simulink model "PECT08"  (R2015b)
settings: Solver=FixedStepAuto  StartTime=0.0  StopTime=100  RelTol=1e-3
undefined symbols (not defined in the file): PDRref, sigbuilder_block
libraries: slrtlib x13, xpcnilib x11, simulink x9, dspfdesign x7, simulink_extras x1
(part 2 of 3)

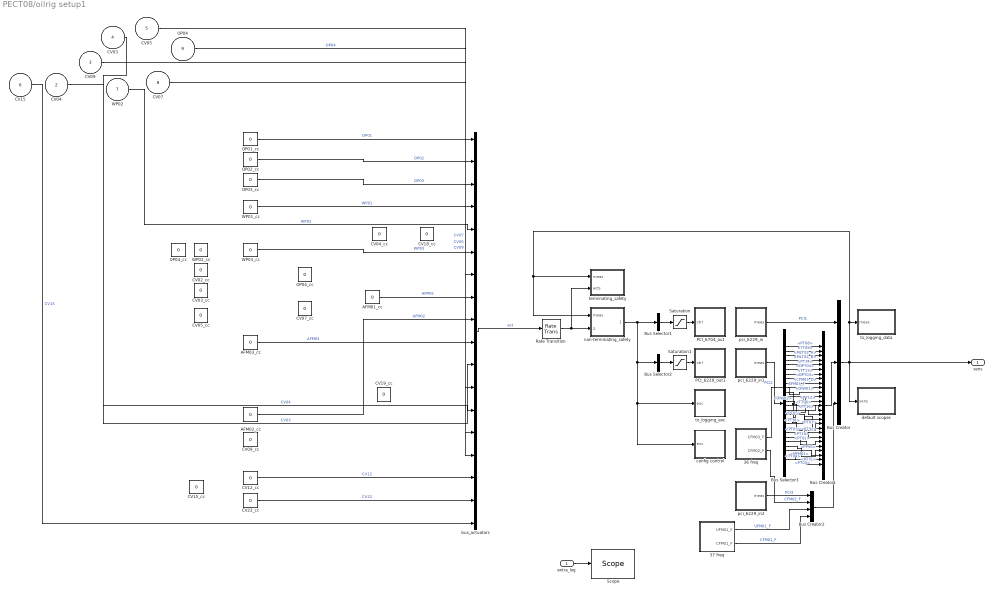
== system PECT08/oilrig setup1 ==
  extra_log : Inport
  CV04 : Inport  Port=2
  CV09 : Inport  Port=3
  CV03 : Inport  Port=4
  CV05 : Inport  Port=5
  CV15 : Inport  Port=6
  WP02 : Inport  Port=7
  CV07 : Inport  Port=8
  OP04 : Inport  Port=9
  0P04_cc : Constant  Value=0
  36 freq : Subsystem  mask{subsystem=[3,6]}
      mask init:
      | sensors = evalin('base','sensors');
      | 
      | subsystem = sprintf('[%d,%d]', subsystem(1), subsystem(2));
      | 
      | freqin = sensors(strcmp(subsystem,{sensors.PCIslot})&(strcmp('FI|0-10000Hz',{sensors.Type})));
      | if ~isempty(freqin)
      |     disp(['PCI slot ' subsystem ' loading']);
      | else
      |     error('There are no frequency inputs in the given card'); 
      | end
  37 freq : Subsystem  mask{subsystem=[3,7]}
      mask init: same as PECT08/oilrig setup1/36 freq
  AFM01_cc : Constant  Value=0
  AFM02_cc : Constant  Value=0
  AFM03_cc : Constant  Value=0
  Bus Creator : BusCreator  Inputs=3
  Bus Creator1 : BusCreator  Inputs=27
  Bus Creator2 : BusCreator  Inputs=4
  Bus Selector1 : BusSelector  OutputSignals=OP01,OP02,OP03,WP01,WP02,OP04,AFM01,AFM02,AFM03,CV03,CV04,CV09,CV05,CV12,CV22,CV15  OutputAsBus=on
  Bus Selector2 : BusSelector  OutputSignals=WP03,CV07  OutputAsBus=on
  Bus Selector3 : BusSelector  OutputSignals=PT08,TT09,MLT02_A,MLT02_B,PT14,DPT04,TT13,DPT03,CFM03_D,OIW01,OIW02,PT12,PT16,TT06,PT05,PT07,PT10,TT11,PT32,TT03,PT15,PT02,PT31,MFM01,PT03,TT04
  CV02_cc : Constant  Value=0
  CV03_cc : Constant  Value=0
  CV04_cc : Constant  Value=0
  CV05_cc : Constant  Value=0
  CV07_cc : Constant  Value=0
  CV09_cc : Constant  Value=0
  CV12_cc : Constant  Value=0
  CV15_cc : Constant  Value=0
  CV18_cc : Constant  Value=0
  CV19_cc : Constant  Value=0
  CV22_cc : Constant  Value=0
  OP01_cc : Constant  Value=0
  OP02_cc : Constant  Value=0
  OP03_cc : Constant  Value=0
  OP04_cc : Constant  Value=0
  PCI_6229_out1 : Subsystem  mask(Actuator output){subsystem=[3,5]}
      mask help: Converts and outputs actuators connected to one PCI-6229 card.
      mask init:
      | %%Get analog channels
      | actuators = evalin('base','actuators');
      | 
      | subsystem = sprintf('[%d,%d]', subsystem(1), subsystem(2));
      | 
      | analogout = actuators(strcmp(subsystem,{actuators.PCIslot}));
      | 
      | src_block = find_system(gcb, 'LookUnderMasks', 'on','Name', 'DA_sink');
      | maskObj = Simulink.Mask.get(src_block{1});
      | 
      | if(isempty(analogout))
      |    error('There are no analog outputs in the given card'); 
      | end
      | 
      | maskObj.Parameters(1,5).Value = subsystem;
      | maskObj.Parameters(1,1).Value = mat2str([analogout.Chan]+1);
      | Simulink.Block.eval(src_block{1});
      | 
      | %Find block
      | transform_blk = find_system(gcb, 'LookUnderMasks', 'on','Name', 'transform');
      | 
      | outputnames = {analogout.ElementName};
      | outputs = strjoin(outputnames,',');
      | 
      | sigcount = numel(outputnames);
      | sigstring = num2str(sigcount);
      | 
      | %Transform block
      | transform_blk = find_system(gcb, 'LookUnderMasks', 'on','Name', 'transform');
      | lines{1}=['function [' outputs ']  = fcn(u,gain,offset)'];
      | lines{2}='   y = u.*gain-offset;';
      | for i=1:numel(outputnames)
      |    %start at 4
      |    lines{2+i} = [ outputnames{i} ' = y(' num2str(i) ');'];
      | end
      | outputscript = strjoin(lines,'\n');
      | matlabfunctionfromstring(transform_blk{1}, outputscript);
      | Simulink.Block.eval(transform_blk{1});
      | 
      | %Delete lines
      | connections = find_system(gcb,'findall','on','LookUnderMasks', 'on','SearchDepth', 1,'type','line');
      | delete_line(connections);
      | 
      | for i=1:numel(outputnames)
      |    add_line(gcb,['transform/' num2str(i) ],['DA_sink/' num2str(i)],'autorouting','on');
      | end
      | 
      | %Transform block
      | add_line(gcb,'ctrl/1','transform/1','autorouting','on')
      | add_line(gcb,'gain/1','transform/2','autorouting','on')
      | add_line(gcb,'offset/1','transform/3','autorouting','on')
      | 
      | gain = [analogout.Gain]';
      | offset = [analogout.Offset]';
      mask DialogControl Control2 Prompt: Subsystem description struct
  PCI_6704_out : Subsystem  mask(Actuator output){subsystem=[3,4]}
      mask help: Converts and outputs actuators connected to one PCI-6229 card.
      mask init:
      | %%Get analog channels
      | actuators = evalin('base','actuators');
      | 
      | subsystem = sprintf('[%d,%d]', subsystem(1), subsystem(2));
      | 
      | analogout = actuators(strcmp(subsystem,{actuators.PCIslot}));
      | 
      | src_block = find_system(gcb, 'LookUnderMasks', 'on','Name', 'DA_sink');
      | maskObj = Simulink.Mask.get(src_block{1});
      | 
      | if(isempty(analogout))
      |    error('There are no analog outputs in the given card'); 
      | end
      | 
      | maskObj.Parameters(1,3).Value = subsystem;
      | maskObj.Parameters(1,1).Value = mat2str([analogout.Chan]+1);
      | Simulink.Block.eval(src_block{1});
      | 
      | %Find block
      | transform_blk = find_system(gcb, 'LookUnderMasks', 'on','Name', 'transform');
      | 
      | outputnames = {analogout.ElementName};
      | outputs = strjoin(outputnames,',');
      | 
      | sigcount = numel(outputnames);
      | sigstring = num2str(sigcount);
      | 
      | %Transform block
      | transform_blk = find_system(gcb, 'LookUnderMasks', 'on','Name', 'transform');
      | lines{1}=['function [' outputs ']  = fcn(u,gain,offset)'];
      | lines{2}='   y = u.*gain-offset;';
      | for i=1:numel(outputnames)
      |    %start at 4
      |    lines{2+i} = [ outputnames{i} ' = y(' num2str(i) ');'];
      | end
      | outputscript = strjoin(lines,'\n');
      | matlabfunctionfromstring(transform_blk{1}, outputscript);
      | Simulink.Block.eval(transform_blk{1});
      | 
      | %Delete lines
      | connections = find_system(gcb,'findall','on','LookUnderMasks', 'on','SearchDepth', 1,'type','line');
      | delete_line(connections);
      | 
      | for i=1:numel(outputnames)
      |    add_line(gcb,['transform/' num2str(i) ],['DA_sink/' num2str(i)],'autorouting','on');
      | end
      | 
      | %Transform block
      | add_line(gcb,'ctrl/1','transform/1','autorouting','on')
      | add_line(gcb,'gain/1','transform/2','autorouting','on')
      | add_line(gcb,'offset/1','transform/3','autorouting','on')
      | 
      | gain = [analogout.Gain]';
      | offset = [analogout.Offset]';
      mask DialogControl Control2 Prompt: Subsystem description struct
  Rate Transition : RateTransition
  Saturation : Saturate  UpperLimit=1  LowerLimit=0
  Saturation1 : Saturate  UpperLimit=1  LowerLimit=0
  "Scope " : slrtlib/Displays and Logging/Scope   scopeno=3  scopetype=Host  autostart=on  viewmode=Graphical sliding  formatstr='%15.6f'  grid=on  ylimits=[1.5,2.5]  nosamples=300  noprepostsamples=0  interleave=1  triggermode=FreeRun  triggersignal=1  trigsignalfromport=off  triggerlevel=0.0  triggerslope=Either  triggerscope=1  triggersample=0  filename=data.dat  mode=Lazy  writesize=512  autorestart=off  dynamicfilemode=off  maxwritefilesize=512*1024^2
  WP01_cc : Constant  Value=0
  WP02_cc : Constant  Value=0
  WP03_cc : Constant  Value=0
  bus_actuators : BusCreator  Inputs=18
  config control : Subsystem
  default scopes : Subsystem
  non-terminating_safety : Subsystem
  pci_6229_in : Subsystem  mask(Sensor reader){subsystem=[3,5]}
      mask help: Reads and converts sensors connected to one PCI-6229 card.
      mask init:
      | %%Get analog channels
      | sensors = evalin('base','sensors');
      | 
      | subsystem = sprintf('[%d,%d]', subsystem(1), subsystem(2));
      | 
      | analogin = sensors(strcmp(subsystem,{sensors.PCIslot})&(strcmp('VI|0-10V',{sensors.Type})|strcmp('VI|2-10V',{sensors.Type})|strcmp('CI|4-20mA',{sensors.Type})));
      | if ~isempty(analogin)
      |     disp(['PCI slot ' subsystem ' loading']);
      | else
      |     error('There are no analog inputs in the given card'); 
      | end
      | 
      | 
      | %%Find source (ADC) block
      | src_block = find_system(gcb, 'LookUnderMasks', 'on','Name', 'src');
      | maskObj = Simulink.Mask.get(src_block{1});
      | 
      | maskObj.Parameters(1,6).Value = subsystem;
      | maskObj.Parameters(1,1).Value = mat2str([analogin.Chan]+1);
      | Simulink.Block.eval(src_block{1});
      | 
      | %Find block
      | transform_blk = find_system(gcb, 'LookUnderMasks', 'on','Name', 'transform');
      | 
      | outputnames = {analogin.ElementName};
      | outputs = strjoin(outputnames,',');
      | 
      | sigcount = numel(outputnames);
      | sigstring = num2str(sigcount);
      | 
      | %Transform block
      | transform_blk = find_system(gcb, 'LookUnderMasks', 'on','Name', 'transform');
      | lines{1}=['function [' outputs ']  = fcn(u,gain,offset)'];
      | lines{2}='   y = u.*gain-offset;';
      | for i=1:numel(outputnames)
      |    %start at 4
      |    lines{2+i} = [ outputnames{i} ' = y(' num2str(i) ');'];
      | end
      | outputscript = strjoin(lines,'\n');
      | matlabfunctionfromstring(transform_blk{1}, outputscript);
      | Simulink.Block.eval(transform_blk{1});
      | 
      | %Delete lines
      | connections = find_system(gcb,'findall','on','LookUnderMasks', 'on','SearchDepth', 1,'type','line');
      | delete_line(connections);
      | 
      | %Mux block
      | mux_blk = find_system(gcb, 'LookUnderMasks', 'on','Name', 'mux');
      | set_param(mux_blk{1},'Inputs', sigstring);
      | Simulink.Block.eval(mux_blk{1});
      | 
      | %Bus block
      | bus_blk = find_system(gcb, 'LookUnderMasks', 'on','Name', 'bus');
      | set_param(bus_blk{1},'Inputs', sigstring);
      | Simulink.Block.eval(bus_blk{1});
      | 
      | for i=1:numel(outputnames)
      |    add_line(gcb,['src/' num2str(i) ],['mux/' num2str(i)],'autorouting','on');
      |    add_line(gcb,['transform/' num2str(i) ],['bus/' num2str(i)],'autorouting','on');
      | end
      | 
      | %Lines to bus block
      | p = get_param(transform_blk, 'PortHandles');
      | l = get_param(p{1}.Outport,'Line');
      | 
      | for i=1:numel(outputnames)
      |    set_param(l{i},'Name',outputnames{i}) 
      | end
      | 
      | %Transform block
      | add_line(gcb,'mux/1','transform/1','autorouting','on')
      | add_line(gcb,'gain/1','transform/2','autorouting','on')
      | add_line(gcb,'offset/1','transform/3','autorouting','on')
      | add_line(gcb,'bus/1','meas/1','autorouting','on')
      | 
      | gain = [analogin.Gain]';
      | offset = [analogin.Offset]';
      mask DialogControl Control2 Prompt: Subsystem description struct
  pci_6229_in1 : Subsystem  mask(Sensor reader){subsystem=[3,6]}
      mask help: Reads and converts sensors connected to one PCI-6229 card.
      mask init:
      | %%Get analog channels
      | sensors = evalin('base','sensors');
      | 
      | subsystem = sprintf('[%d,%d]', subsystem(1), subsystem(2));
      | 
      | freqin = sensors(strcmp(subsystem,{sensors.PCIslot})&(strcmp('FI|0-10000Hz',{sensors.Type})));
      | if ~isempty(freqin)
      |     disp(['PCI slot ' subsystem ' loading']);
      | else
      |     error('There are no frequency inputs in the given card'); 
      | end
      | 
      | analogin = sensors(strcmp(subsystem,{sensors.PCIslot})&(strcmp('VI|0-10V',{sensors.Type})|strcmp('VI|2-10V',{sensors.Type})|strcmp('CI|4-20mA',{sensors.Type})));
      | if ~isempty(analogin)
      |     disp(['PCI slot ' subsystem ' loading']);
      | else
      |     error('There are no analog inputs in the given card'); 
      | end
      | 
      | 
      | %%Find source (ADC) block
      | src_block = find_system(gcb, 'LookUnderMasks', 'on','Name', 'src');
      | maskObj = Simulink.Mask.get(src_block{1});
      | 
      | maskObj.Parameters(1,6).Value = subsystem;
      | maskObj.Parameters(1,1).Value = mat2str([analogin.Chan]+1);
      | Simulink.Block.eval(src_block{1});
      | 
      | %Find block
      | transform_blk = find_system(gcb, 'LookUnderMasks', 'on','Name', 'transform');
      | 
      | outputnames = {analogin.ElementName};
      | outputs = strjoin(outputnames,',');
      | 
      | sigcount = numel(outputnames);
      | sigstring = num2str(sigcount);
      | 
      | %Transform block
      | transform_blk = find_system(gcb, 'LookUnderMasks', 'on','Name', 'transform');
      | lines{1}=['function [' outputs ']  = fcn(u,gain,offset)'];
      | lines{2}='   y = u.*gain-offset;';
      | for i=1:numel(outputnames)
      |    %start at 4
      |    lines{2+i} = [ outputnames{i} ' = y(' num2str(i) ');'];
      | end
      | outputscript = strjoin(lines,'\n');
      | matlabfunctionfromstring(transform_blk{1}, outputscript);
      | Simulink.Block.eval(transform_blk{1});
      | 
      | %Delete lines
      | connections = find_system(gcb,'findall','on','LookUnderMasks', 'on','SearchDepth', 1,'type','line');
      | delete_line(connections);
      | 
      | %Mux block
      | mux_blk = find_system(gcb, 'LookUnderMasks', 'on','Name', 'mux');
      | set_param(mux_blk{1},'Inputs', sigstring);
      | Simulink.Block.eval(mux_blk{1});
      | 
      | %Bus block
      | bus_blk = find_system(gcb, 'LookUnderMasks', 'on','Name', 'bus');
      | set_param(bus_blk{1},'Inputs', sigstring);
      | Simulink.Block.eval(bus_blk{1});
      | 
      | for i=1:numel(outputnames)
      |    add_line(gcb,['src/' num2str(i) ],['mux/' num2str(i)],'autorouting','on');
      |    add_line(gcb,['transform/' num2str(i) ],['bus/' num2str(i)],'autorouting','on');
      | end
      | 
      | %Lines to bus block
      | p = get_param(transform_blk, 'PortHandles');
      | l = get_param(p{1}.Outport,'Line');
      | 
      | for i=1:numel(outputnames)
      |    set_param(l{i},'Name',outputnames{i}) 
      | end
      | 
      | %Transform block
      | add_line(gcb,'mux/1','transform/1','autorouting','on')
      | add_line(gcb,'gain/1','transform/2','autorouting','on')
      | add_line(gcb,'offset/1','transform/3','autorouting','on')
      | add_line(gcb,'bus/1','meas/1','autorouting','on')
      | 
      | gain = [analogin.Gain]';
      | offset = [analogin.Offset]';
      mask DialogControl Control2 Prompt: Subsystem description struct
  pci_6229_in2 : Subsystem  mask(Sensor reader){subsystem=[3,7]}
      mask help: Reads and converts sensors connected to one PCI-6229 card.
      mask init:
      | %%Get analog channels
      | sensors = evalin('base','sensors');
      | 
      | subsystem = sprintf('[%d,%d]', subsystem(1), subsystem(2));
      | 
      | analogin = sensors(strcmp(subsystem,{sensors.PCIslot})&(strcmp('VI|0-10V',{sensors.Type})|strcmp('VI|2-10V',{sensors.Type})|strcmp('CI|4-20mA',{sensors.Type})));
      | if ~isempty(analogin)
      |     disp(['PCI slot ' subsystem ' loading']);
      | else
      |     error('There are no analog inputs in the given card'); 
      | end
      | 
      | freqin = sensors(strcmp(subsystem,{sensors.PCIslot})&(strcmp('FI|0-10000Hz',{sensors.Type})));
      | if ~isempty(freqin)
      |     disp(['PCI slot ' subsystem ' loading']);
      | else
      |     error('There are no analog inputs in the given card'); 
      | end
      | 
      | 
      | 
      | %%Find source (ADC) block
      | src_block = find_system(gcb, 'LookUnderMasks', 'on','Name', 'src');
      | maskObj = Simulink.Mask.get(src_block{1});
      | 
      | maskObj.Parameters(1,6).Value = subsystem;
      | maskObj.Parameters(1,1).Value = mat2str([analogin.Chan]+1);
      | Simulink.Block.eval(src_block{1});
      | 
      | %Find block
      | transform_blk = find_system(gcb, 'LookUnderMasks', 'on','Name', 'transform');
      | 
      | outputnames = {analogin.ElementName};
      | outputs = strjoin(outputnames,',');
      | 
      | sigcount = numel(outputnames);
      | sigstring = num2str(sigcount);
      | 
      | %Transform block
      | transform_blk = find_system(gcb, 'LookUnderMasks', 'on','Name', 'transform');
      | lines{1}=['function [' outputs ']  = fcn(u,gain,offset)'];
      | lines{2}='   y = u.*gain-offset;';
      | for i=1:numel(outputnames)
      |    %start at 4
      |    lines{2+i} = [ outputnames{i} ' = y(' num2str(i) ');'];
      | end
      | outputscript = strjoin(lines,'\n');
      | matlabfunctionfromstring(transform_blk{1}, outputscript);
      | Simulink.Block.eval(transform_blk{1});
      | 
      | %Delete lines
      | connections = find_system(gcb,'findall','on','LookUnderMasks', 'on','SearchDepth', 1,'type','line');
      | delete_line(connections);
      | 
      | %Mux block
      | mux_blk = find_system(gcb, 'LookUnderMasks', 'on','Name', 'mux');
      | set_param(mux_blk{1},'Inputs', sigstring);
      | Simulink.Block.eval(mux_blk{1});
      | 
      | %Bus block
      | bus_blk = find_system(gcb, 'LookUnderMasks', 'on','Name', 'bus');
      | set_param(bus_blk{1},'Inputs', sigstring);
      | Simulink.Block.eval(bus_blk{1});
      | 
      | for i=1:numel(outputnames)
      |    add_line(gcb,['src/' num2str(i) ],['mux/' num2str(i)],'autorouting','on');
      |    add_line(gcb,['transform/' num2str(i) ],['bus/' num2str(i)],'autorouting','on');
      | end
      | 
      | %Lines to bus block
      | p = get_param(transform_blk, 'PortHandles');
      | l = get_param(p{1}.Outport,'Line');
      | 
      | for i=1:numel(outputnames)
      |    set_param(l{i},'Name',outputnames{i}) 
      | end
      | 
      | %Transform block
      | add_line(gcb,'mux/1','transform/1','autorouting','on')
      | add_line(gcb,'gain/1','transform/2','autorouting','on')
      | add_line(gcb,'offset/1','transform/3','autorouting','on')
      | add_line(gcb,'bus/1','meas/1','autorouting','on')
      | 
      | gain = [analogin.Gain]';
      | offset = [analogin.Offset]';
      mask DialogControl Control2 Prompt: Subsystem description struct
  terminating_safety : Subsystem
  to_logging_data : Subsystem
  to_logging_exc : Subsystem
  sens : Outport
  wires:
  non-terminating_safety/1(acts_out) -> config control/1(exc), to_logging_exc/1(exc), Bus Selector2/1, Bus Selector1/1
  pci_6229_in/1(meas) -> Bus Creator/1  "PCI1"
  Bus Selector3/2 -> Bus Creator1/2  "<TT09>"
  Bus Selector3/3 -> Bus Creator1/3  "<MLT02_A>"
  Bus Selector3/9 -> Bus Creator1/9  "<CFM03_D>"
  Bus Selector3/24 -> Bus Creator1/25  "<MFM01>"
  Bus Selector3/25 -> Bus Creator1/26  "<PT03>"
  Bus Selector3/21 -> Bus Creator1/22  "<PT15>"
  pci_6229_in2/1(meas) -> Bus Creator2/1  "PCI3"
  bus_actuators/1 -> Rate Transition/1  "act"
  Rate Transition/1 -> terminating_safety/2(acts), non-terminating_safety/2(acts_in)
  Bus Selector1/1 -> Saturation/1
  Bus Selector3/4 -> Bus Creator1/4  "<MLT02_B>"
  Bus Selector3/14 -> Bus Creator1/15  "<TT06>"
  Bus Selector3/26 -> Bus Creator1/27  "<TT04>"
  Bus Selector3/23 -> Bus Creator1/24  "<PT31>"
  Bus Selector3/16 -> Bus Creator1/17  "<PT07>"
  Bus Selector3/22 -> Bus Creator1/23  "<PT02>"
  Bus Selector3/20 -> Bus Creator1/21  "<TT03>"
  Bus Selector3/18 -> Bus Creator1/19  "<TT11>"
  Bus Selector2/1 -> Saturation1/1
  pci_6229_in1/1(meas) -> Bus Selector3/1  "PCI2"
  Bus Selector3/1 -> Bus Creator1/1  "<PT08>"
  Bus Selector3/5 -> Bus Creator1/5  "<PT14>"
  Bus Selector3/7 -> Bus Creator1/7  "<TT13>"
  Bus Selector3/19 -> Bus Creator1/20  "<PT32>"
  Bus Selector3/6 -> Bus Creator1/6  "<DPT04>"
  37 freq/1(UFM01_F) -> Bus Creator2/3  "UFM01_F"
  Bus Selector3/17 -> Bus Creator1/18  "<PT10>"
  Bus Selector3/8 -> Bus Creator1/8  "<DPT03>"
  Bus Creator1/1 -> Bus Creator/2
  Bus Selector3/13 -> Bus Creator1/14  "<PT16>"
  Bus Creator/1 -> sens/1, non-terminating_safety/1(meas), terminating_safety/1(meas), to_logging_data/1(meas), default scopes/1(sens)
  36 freq/1(CFM03_F) -> Bus Creator1/10  "CFM03_F"
  Bus Selector3/15 -> Bus Creator1/16  "<PT05>"
  36 freq/2(CFM02_F) -> Bus Creator2/2  "CFM02_F"
  Saturation1/1 -> PCI_6229_out1/1(ctrl)
  Saturation/1 -> PCI_6704_out/1(ctrl)
  Bus Creator2/1 -> Bus Creator/3
  37 freq/2(CFM01_F) -> Bus Creator2/4  "CFM01_F"
  extra_log/1 -> "Scope "/1
  Bus Selector3/12 -> Bus Creator1/13  "<PT12>"
  Bus Selector3/10 -> Bus Creator1/11  "<OIW01>"
  Bus Selector3/11 -> Bus Creator1/12  "<OIW02>"
  OP01_cc/1 -> bus_actuators/1  "OP01"
  OP02_cc/1 -> bus_actuators/2  "OP02"
  OP03_cc/1 -> bus_actuators/3  "OP03"
  WP01_cc/1 -> bus_actuators/4  "WP01"
  WP02/1 -> bus_actuators/5  "WP02"
  WP03_cc/1 -> bus_actuators/6  "WP03"
  OP04/1 -> bus_actuators/7  "OP04"
  AFM01_cc/1 -> bus_actuators/8  "AFM01"
  AFM02_cc/1 -> bus_actuators/9  "AFM02"
  AFM03_cc/1 -> bus_actuators/10  "AFM03"
  CV03/1 -> bus_actuators/11  "CV03"
  CV07/1 -> bus_actuators/12  "CV07"
  CV04/1 -> bus_actuators/13  "CV04"
  CV09/1 -> bus_actuators/14  "CV09"
  CV05/1 -> bus_actuators/15  "CV05"
  CV12_cc/1 -> bus_actuators/16  "CV12"
  CV22_cc/1 -> bus_actuators/17  "CV22"
  CV15/1 -> bus_actuators/18  "CV15"

== system PECT08/Subsystem/Fi ==
  Demux : Demux  Tag=STV Demux  Outputs=1
  FromWs : FromWorkspace  Tag=STV FromWs  VariableName=tuvar  SampleTime=0
      SigBuilderData=|
      | common.afterFinalStr = 'Extrapolate'
      | common.sampleTime = 0
      | dataSet.timeRange = [0 1000]
      | dataSet.name = 'Group 1'
      | sbobj.Groups.Name = 'Group 1'
      | sbobj.Groups.Signals.Name = 'Signal 1'
      | sbobj.Groups.Signals.XData = [0 100 100 150 150 200 200 250 250 300 300 350 350 400 400 450 450 550 550 1000]
      | sbobj.Groups.Signals.YData = [0.37 0.37 0.45 0.45 0.536 0.536 0.4 0.4 0.65 0.65 0.6 0.6 0.37 0.37 0.7 0.7 0.6 0.6 0.4 0.4]
      | sbobj.Groups.TimeRange = [0 1000]
  Signal 1 : Outport  Tag=STV Outport
  wires:
  Demux/1 -> Signal 1/1
  FromWs/1 -> Demux/1

== system PECT08/Subsystem/Flow_oscilation ==
  Demux : Demux  Tag=STV Demux  Outputs=1
  FromWs : FromWorkspace  Tag=STV FromWs  VariableName=tuvar  SampleTime=0
      SigBuilderData=|
      | common.afterFinalStr = 'Extrapolate'
      | common.sampleTime = 0
      | dataSet.timeRange = [0 1000]
      | dataSet.name = 'Group 1'
      | sbobj.Groups.Name = 'Group 1'
      | sbobj.Groups.Signals.Name = 'Signal 1'
      | sbobj.Groups.Signals.XData = [0 20 40 60 80 100 120 140 160 180 200 220 240 260 280 300 320 340 360 380 400 420 440 460 480 500 520 540 560 580 600 620 640 660 680 700 720 740 760 780 800 820 840 860 880 900 920 940 960 980 1000]
      | sbobj.Groups.Signals.YData = [0.591075140817 0.64106188151 0.609589965532 0.644005700352 0.643757231826 0.53255913549 0.566918274019 0.562359456094 0.636073779882 0.678808051234 0.606927430849 0.652492920186 0.641821604141 0.577934707619 0.635898679832 0.589924210453 0.680650675866 0.618697339632 0.685439986291 0.602997660376 0.643577334669 0.617488350971 0.539121642798 0.580714738969 0.644500451927 0.6178045548 0.575250719902 0.594944858445 0.629980709623 0.580279239738 0.658998008992 0.594371619731 0.692354504821 0.57680534997 0.627967577763 0.559158937529 0.591054754988 0.5962699874 0.636053453593 0.657685332769 0.632019438704 0.605077173655 0.652619540324 0.651955479686 0.624808211278 0.642849905189 0.636511840412 0.580521524666 0.650382733037 0.593711948036 0.595843260745]
      | sbobj.Groups.TimeRange = [0 1000]
  Signal 1 : Outport  Tag=STV Outport
  wires:
  Demux/1 -> Signal 1/1
  FromWs/1 -> Demux/1

== system PECT08/Subsystem/Flow_oscilation1 ==
  Demux : Demux  Tag=STV Demux  Outputs=1
  FromWs : FromWorkspace  Tag=STV FromWs  VariableName=tuvar  SampleTime=0
      SigBuilderData=|
      | common.afterFinalStr = 'Extrapolate'
      | common.sampleTime = 0
      | dataSet.timeRange = [0 1000]
      | dataSet.name = 'Group 1'
      | sbobj.Groups.Name = 'Group 1'
      | sbobj.Groups.Signals.Name = 'Signal 1'
      | sbobj.Groups.Signals.XData = [0 4.16666666667 8.33333333333 12.5 16.6666666667 20.8333333333 25 29.1666666667 33.3333333333 37.5 41.6666666667 45.8333333333 ... (241 elements, 1x241)]
      | sbobj.Groups.Signals.YData = [0.6 0.635355339059 0.65 0.635355339059 0.6 0.564644660941 0.55 0.564644660941 0.6 0.635355339059 0.65 0.635355339059 ... (241 elements, 1x241)]
      | sbobj.Groups.TimeRange = [0 1000]
  Signal 1 : Outport  Tag=STV Outport
  wires:
  Demux/1 -> Signal 1/1
  FromWs/1 -> Demux/1

== system PECT08/Subsystem/Flow_oscilation2 ==
  Demux : Demux  Tag=STV Demux  Outputs=3
  FromWs : FromWorkspace  Tag=STV FromWs  VariableName=tuvar  SampleTime=0
      SigBuilderData=|
      | common.afterFinalStr = 'Extrapolate'
      | common.sampleTime = 0
      | dataSet.timeRange = [0 1550]
      | dataSet.name = 'Group 1'
      | sbobj.Groups.Name = 'Group 1'
      | sbobj.Groups.Signals(1).Name = 'CV09'
      | sbobj.Groups.Signals(1).XData = [0 50 50 100 100 150 150 200 200 250 250 300 300 350 350 400 400 450 450 500 500 550 550 600 600 650 650 700 700 750 750 800 800 850 850 900 900 950 950 1000 1000 1050 1050 1100 1100 1150 1150 1200 1200 1250 1250 1300 1300 1350 1350 1400 1400 1450 1450 1500 1550]
      | sbobj.Groups.Signals(1).YData = [0 1 0 1 0 1 0 1 0 1 0 1 0 1 0 1 0 1 0 1 0 1 0 1 0 1 0 1 0 1 0 1 0 1 0 1 0 1 0 1 0 1 0 1 0 1 0 1 0 1 0 1 0 1 0 1 0 1 0 1 1]
      | sbobj.Groups.Signals(2).Name = 'Signal 1'
      | sbobj.Groups.Signals(2).XData = [0 66.6666666667 66.6666666667 133.333333333 133.333333333 200 200 266.666666667 266.666666667 333.333333333 333.333333333 400 400 466.666666667 466.666666667 533.333333333 533.333333333 600 600 666.666666667 666.666666667 733.333333333 733.333333333 800 800 866.666666667 866.666666667 933.333333333 933.333333333 1000 1000 1066.66666667 1066.66666667 1133.33333333 1133.33333333 1200 1200 1266.66666667 1266.66666667 1333.33333333 1333.33333333 1400 1400 1466.66666667 1466.66666667 1500 1550]
      | sbobj.Groups.Signals(2).YData = [0 1 0 1 0 1 0 1 0 1 0 1 0 1 0 1 0 1 0 1 0 1 0 1 0 1 0 1 0 1 0 1 0 1 0 1 0 1 0 1 0 1 0 1 0 0.5 0.5]
      | sbobj.Groups.Signals(3).Name = 'Signal 2'
      | sbobj.Groups.Signals(3).XData = [0 66.6666666667 66.6666666667 133.333333333 133.333333333 200 200 266.666666667 266.666666667 333.333333333 333.333333333 400 400 466.666666667 466.666666667 533.333333333 533.333333333 600 600 666.666666667 666.666666667 733.333333333 733.333333333 800 800 866.666666667 866.666666667 933.333333333 933.333333333 1000 1000 1066.66666667 1066.66666667 1133.33333333 1133.33333333 1200 1200 1266.66666667 1266.66666667 1333.33333333 1333.33333333 1400 1400 1466.66666667 1466.66666667 1533.33333333 1533.33333333 1550]
      | sbobj.Groups.Signals(3).YData = [0 1 0 1 0 1 0 1 0 1 0 1 0 1 0 1 0 1 0 1 0 1 0 1 0 1 0 1 0 1 0 1 0 1 0 1 0 1 0 1 0 1 0 1 0 1 0 0.25]
      | sbobj.Groups.TimeRange = [0 1550]
  CV09 : Outport  Tag=STV Outport
  Signal 1 : Outport  Tag=STV Outport  Port=2
  Signal 2 : Outport  Tag=STV Outport  Port=3
  wires:
  FromWs/1 -> Demux/1
  Demux/1 -> CV09/1
  Demux/2 -> Signal 1/1
  Demux/3 -> Signal 2/1

== system PECT08/Subsystem/Flow_oscilation3 ==
  Demux : Demux  Tag=STV Demux  Outputs=1
  FromWs : FromWorkspace  Tag=STV FromWs  VariableName=tuvar  SampleTime=0
      SigBuilderData=|
      | common.afterFinalStr = 'Extrapolate'
      | common.sampleTime = 0
      | dataSet.timeRange = [0 1000]
      | dataSet.name = 'Group 1'
      | sbobj.Groups.Name = 'Group 1'
      | sbobj.Groups.Signals.Name = 'CV09'
      | sbobj.Groups.Signals.XData = [0 6.25 12.5 18.75 25 31.25 37.5 43.75 50 56.25 62.5 68.75 75 81.25 87.5 93.75 100 106.25 112.5 118.75 125 131.25 137.5 143.75 150 156.25 162.5 168.75 175 181.25 187.5 193.75 200 206.25 212.5 218.75 225 231.25 237.5 243.75 250 256.25 262.5 268.75 275 281.25 287.5 293.75 300 306.25 312.5 318.75 325 331.25 337.5 343.75 350 356.25 362.5 368.75 375 381.25 387.5 393.75 400 406.25 412.5 418.75 425 431.25 437.5 443.75 450 456.25 462.5 468.75 475 481.25 487.5 493.75 500 506.25 512.5 518.75 525 531.25 537.5 543.75 550 556.25 562.5 568.75 575 581.25 587.5 593.75 600 606.25 612.5 618.75 625 631.25 637.5 643.75 650 656.25 662.5 668.75 675 681.25 687.5 693.75 700 706.25 712.5 718.75 725 731.25 737.5 743.75 750 756.25 762.5 768.75 775 781.25 787.5 793.75 800 806.25 812.5 818.75 825 831.25 837.5 843.75 850 856.25 862.5 868.75 875 881.25 887.5 893.75 900 906.25 912.5 918.75 925 931.25 937.5 943.75 950 956.25 962.5 968.75 975 981.25 987.5 993.75 1000]
      | sbobj.Groups.Signals.YData = [0.5 0.853553390593 1 0.853553390593 0.5 0.146446609407 0 0.146446609407 0.5 0.853553390593 1 0.853553390593 0.5 0.146446609407 0 0.146446609407 0.5 0.853553390593 1 0.853553390593 0.5 0.146446609407 0 0.146446609407 0.5 0.853553390593 1 0.853553390593 0.5 0.146446609407 0 0.146446609407 0.5 0.853553390593 1 0.853553390593 0.5 0.146446609407 0 0.146446609407 0.5 0.853553390593 1 0.853553390593 0.5 0.146446609407 0 0.146446609407 0.5 0.853553390593 1 0.853553390593 0.5 0.146446609407 0 0.146446609407 0.5 0.853553390593 1 0.853553390593 0.5 0.146446609407 0 0.146446609407 0.5 0.853553390593 1 0.853553390593 0.5 0.146446609407 0 0.146446609407 0.5 0.853553390593 1 0.853553390593 0.5 0.146446609407 0 0.146446609407 0.5 0.853553390593 1 0.853553390593 0.5 0.146446609407 0 0.146446609407 0.5 0.853553390593 1 0.853553390593 0.5 0.146446609407 0 0.146446609407 0.5 0.853553390593 1 0.853553390593 0.5 0.146446609407 0 0.146446609407 0.5 0.853553390593 1 0.853553390593 0.5 0.146446609407 0 0.146446609407 0.5 0.853553390593 1 0.853553390593 0.5 0.146446609407 0 0.146446609407 0.5 0.853553390593 1 0.853553390593 0.5 0.146446609407 0 0.146446609407 0.5 0.853553390593 1 0.853553390593 0.5 0.146446609407 0 0.146446609407 0.5 0.853553390593 1 0.853553390593 0.5 0.146446609407 0 0.146446609407 0.5 0.853553390593 1 0.853553390593 0.5 0.146446609407 0 0.146446609407 0.5 0.853553390593 1 0.853553390593 0.5 0.146446609407 0 0.146446609407 0.5]
      | sbobj.Groups.TimeRange = [0 1000]
  CV09 : Outport  Tag=STV Outport
  wires:
  FromWs/1 -> Demux/1
  Demux/1 -> CV09/1

== system PECT08/Subsystem/Flow_slug_Triangle ==
  Demux : Demux  Tag=STV Demux  Outputs=1
  FromWs : FromWorkspace  Tag=STV FromWs  VariableName=tuvar  SampleTime=0
      SigBuilderData=|
      | common.afterFinalStr = 'Extrapolate'
      | common.sampleTime = 0
      | dataSet.timeRange = [0 500]
      | dataSet.name = 'Group 1'
      | sbobj.Groups.Name = 'Group 1'
      | sbobj.Groups.Signals.Name = 'Signal 1'
      | sbobj.Groups.Signals.XData = [0 20 40 60 60 80 80 100 100 120 120 140 140 160 160 180 180 200 200 220 220 240 240 260 260 280 280 300 300 320 320 340 340 360 360 380 380 400 400 420 420 440 440 460 460 480 480 500]
      | sbobj.Groups.Signals.YData = [0.7 0.7 0.7 0.7 0.2 0.7 0.2 0.7 0.2 0.7 0.2 0.7 0.2 0.7 0.2 0.7 0.2 0.7 0.2 0.7 0.2 0.7 0.2 0.7 0.2 0.7 0.2 0.7 0.2 0.7 0.2 0.7 0.2 0.7 0.2 0.7 0.2 0.7 0.2 0.7 0.2 0.7 0.2 0.7 0.2 0.7 0.2 0.7]
      | sbobj.Groups.TimeRange = [0 500]
  Signal 1 : Outport  Tag=STV Outport
  wires:
  Demux/1 -> Signal 1/1
  FromWs/1 -> Demux/1

== system PECT08/Subsystem/Flow_slug_square ==
  Demux : Demux  Tag=STV Demux  Outputs=1
  FromWs : FromWorkspace  Tag=STV FromWs  VariableName=tuvar  SampleTime=0
      SigBuilderData=|
      | common.afterFinalStr = 'Extrapolate'
      | common.sampleTime = 0
      | dataSet.timeRange = [0 500]
      | dataSet.name = 'Group 1'
      | sbobj.Groups.Name = 'Group 1'
      | sbobj.Groups.Signals.Name = 'Signal 1'
      | sbobj.Groups.Signals.XData = [0 10 20 30 40 50 50 60 60 70 70 80 80 90 90 100 100 110 110 120 120 130 130 140 140 150 150 160 160 170 170 180 180 190 190 200 200 210 210 220 220 230 230 240 240 250 250 260 260 270 270 280 280 290 290 300 300 310 310 320 320 330 330 340 340 350 350 360 360 370 370 380 380 390 390 400 400 410 410 420 420 430 430 440 440 450 450 460 460 470 470 480 480 490 490 500]
      | sbobj.Groups.Signals.YData = [0.7 0.7 0.7 0.7 0.7 0.7 0.2 0.2 0.7 0.7 0.2 0.2 0.7 0.7 0.2 0.2 0.7 0.7 0.2 0.2 0.7 0.7 0.2 0.2 0.7 0.7 0.2 0.2 0.7 0.7 0.2 0.2 0.7 0.7 0.2 0.2 0.7 0.7 0.2 0.2 0.7 0.7 0.2 0.2 0.7 0.7 0.2 0.2 0.7 0.7 0.2 0.2 0.7 0.7 0.2 0.2 0.7 0.7 0.2 0.2 0.7 0.7 0.2 0.2 0.7 0.7 0.2 0.2 0.7 0.7 0.2 0.2 0.7 0.7 0.2 0.2 0.7 0.7 0.2 0.2 0.7 0.7 0.2 0.2 0.7 0.7 0.2 0.2 0.7 0.7 0.2 0.2 0.7 0.7 0.2 0.2]
      | sbobj.Groups.TimeRange = [0 500]
  Signal 1 : Outport  Tag=STV Outport
  wires:
  Demux/1 -> Signal 1/1
  FromWs/1 -> Demux/1

== system PECT08/Subsystem/Flow_slug_square_long ==
  Demux : Demux  Tag=STV Demux  Outputs=1
  FromWs : FromWorkspace  Tag=STV FromWs  VariableName=tuvar  SampleTime=0
      SigBuilderData=|
      | common.afterFinalStr = 'Extrapolate'
      | common.sampleTime = 0
      | dataSet.timeRange = [0 1000]
      | dataSet.name = 'Group 1'
      | sbobj.Groups.Name = 'Group 1'
      | sbobj.Groups.Signals.Name = 'Signal 1'
      | sbobj.Groups.Signals.XData = [0 16.6666666667 33.3333333333 50 50 66.6666666667 66.6666666667 83.3333333333 83.3333333333 100 100 116.666666667 116.666666667 133.333333333 133.333333333 150 150 166.666666667 166.666666667 183.333333333 183.333333333 200 200 216.666666667 216.666666667 233.333333333 233.333333333 250 250 266.666666667 266.666666667 283.333333333 283.333333333 300 300 316.666666667 316.666666667 333.333333333 333.333333333 350 350 366.666666667 366.666666667 383.333333333 383.333333333 400 400 416.666666667 416.666666667 433.333333333 433.333333333 450 450 466.666666667 466.666666667 483.333333333 483.333333333 500 500 516.666666667 516.666666667 533.333333333 533.333333333 550 550 566.666666667 566.666666667 583.333333333 583.333333333 600 600 616.666666667 616.666666667 633.333333333 633.333333333 650 650 666.666666667 666.666666667 683.333333333 683.333333333 700 700 716.666666667 716.666666667 733.333333333 733.333333333 750 750 766.666666667 766.666666667 783.333333333 783.333333333 800 800 816.666666667 816.666666667 833.333333333 833.333333333 850 850 866.666666667 866.666666667 883.333333333 883.333333333 900 900 916.666666667 916.666666667 933.333333333 933.333333333 950 950 966.666666667 966.666666667 983.333333333 983.333333333 1000]
      | sbobj.Groups.Signals.YData = [0.7 0.7 0.7 0.7 0.2 0.2 0.7 0.7 0.2 0.2 0.7 0.7 0.2 0.2 0.7 0.7 0.2 0.2 0.7 0.7 0.2 0.2 0.7 0.7 0.2 0.2 0.7 0.7 0.2 0.2 0.7 0.7 0.2 0.2 0.7 0.7 0.2 0.2 0.7 0.7 0.2 0.2 0.7 0.7 0.2 0.2 0.7 0.7 0.2 0.2 0.7 0.7 0.2 0.2 0.7 0.7 0.2 0.2 0.7 0.7 0.2 0.2 0.7 0.7 0.2 0.2 0.7 0.7 0.2 0.2 0.7 0.7 0.2 0.2 0.7 0.7 0.2 0.2 0.7 0.7 0.2 0.2 0.7 0.7 0.2 0.2 0.7 0.7 0.2 0.2 0.7 0.7 0.2 0.2 0.7 0.7 0.2 0.2 0.7 0.7 0.2 0.2 0.7 0.7 0.2 0.2 0.7 0.7 0.2 0.2 0.7 0.7 0.2 0.2 0.7 0.7 0.2 0.7]
      | sbobj.Groups.TimeRange = [0 1000]
  Signal 1 : Outport  Tag=STV Outport
  wires:
  Demux/1 -> Signal 1/1
  FromWs/1 -> Demux/1

== system PECT08/Subsystem/Flow_step  ==
  Demux : Demux  Tag=STV Demux  Outputs=1
  FromWs : FromWorkspace  Tag=STV FromWs  VariableName=tuvar  SampleTime=0
      SigBuilderData=|
      | common.afterFinalStr = 'Extrapolate'
      | common.sampleTime = 0
      | dataSet.timeRange = [0 1000]
      | dataSet.name = 'Group 1'
      | sbobj.Groups.Name = 'Group 1'
      | sbobj.Groups.Signals.Name = 'Signal 1'
      | sbobj.Groups.Signals.XData = [0 100 100 150 150 200 200 250 250 1000]
      | sbobj.Groups.Signals.YData = [0.7 0.7 0.5 0.5 0.7 0.7 0.3 0.3 0.5 0.5]
      | sbobj.Groups.TimeRange = [0 1000]
  Signal 1 : Outport  Tag=STV Outport
  wires:
  Demux/1 -> Signal 1/1
  FromWs/1 -> Demux/1

== system PECT08/Subsystem/Signal Builder ==
  Demux : Demux  Tag=STV Demux  Outputs=1
  FromWs : FromWorkspace  Tag=STV FromWs  VariableName=tuvar  SampleTime=0
      SigBuilderData=|
      | common.afterFinalStr = 'Extrapolate'
      | common.sampleTime = 0
      | dataSet.timeRange = [0 1000]
      | dataSet.name = 'Group 1'
      | sbobj.Groups.Name = 'Group 1'
      | sbobj.Groups.Signals.Name = 'PDR_Reference'
      | sbobj.Groups.Signals.XData = [0 100 100 150 150 200 200 250 250 300 300 350 350 1000]
      | sbobj.Groups.Signals.YData = [1.7 1.7 2.3 2.3 1.5 1.5 2 2 2.5 2.5 1.7 1.7 2 2]
      | sbobj.Groups.TimeRange = [0 1000]
  PDR_Reference : Outport  Tag=STV Outport
  wires:
  Demux/1 -> PDR_Reference/1
  FromWs/1 -> Demux/1

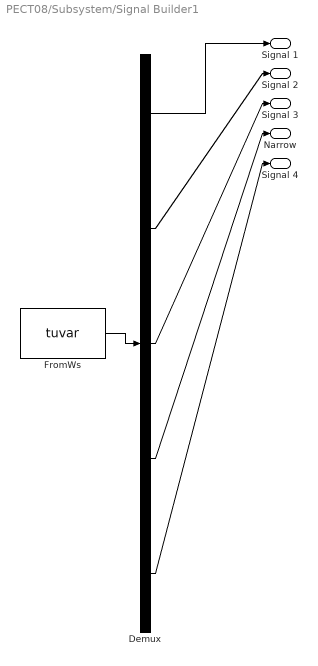
== system PECT08/Subsystem/Signal Builder1 ==
  Demux : Demux  Tag=STV Demux  Outputs=5
  FromWs : FromWorkspace  Tag=STV FromWs  VariableName=tuvar  SampleTime=0
      SigBuilderData=|
      | common.afterFinalStr = 'Extrapolate'
      | common.sampleTime = 0
      | dataSet.timeRange = [0 1550]
      | dataSet.name = 'Group 1'
      | sbobj.Groups.Name = 'Group 1'
      | sbobj.Groups.Signals(1).Name = 'Signal 1'
      | sbobj.Groups.Signals(1).XData = [0 1550]
      | sbobj.Groups.Signals(1).YData = [2.3 2.3]
      | sbobj.Groups.Signals(2).Name = 'Signal 2'
      | sbobj.Groups.Signals(2).XData = [0 100 500 600 1000 1550]
      | sbobj.Groups.Signals(2).YData = [1 1 0.4 0.4 1 1]
      | sbobj.Groups.Signals(3).Name = 'Signal 3'
      | sbobj.Groups.Signals(3).XData = [0 100 500 600 1000 1550]
      | sbobj.Groups.Signals(3).YData = [0.2 0.2 0.7 0.7 0.2 0.2]
      | sbobj.Groups.Signals(4).Name = 'Narrow'
      | sbobj.Groups.Signals(4).XData = [0 100 500 600 1000 1550]
      | sbobj.Groups.Signals(4).YData = [0.45 0.45 0.36 0.36 0.45 0.45]
      | sbobj.Groups.Signals(5).Name = 'Signal 4'
      | sbobj.Groups.Signals(5).XData = [0 100 1450 1550]
      | sbobj.Groups.Signals(5).YData = [1 1 0.36 0.36]
      | sbobj.Groups.TimeRange = [0 1550]
  Signal 1 : Outport  Tag=STV Outport
  Signal 2 : Outport  Tag=STV Outport  Port=2
  Signal 3 : Outport  Tag=STV Outport  Port=3
  Narrow : Outport  Tag=STV Outport  Port=4
  Signal 4 : Outport  Tag=STV Outport  Port=5
  wires:
  Demux/1 -> Signal 1/1
  FromWs/1 -> Demux/1
  Demux/2 -> Signal 2/1
  Demux/3 -> Signal 3/1
  Demux/4 -> Narrow/1
  Demux/5 -> Signal 4/1

== system PECT08/Subsystem/Signal Builder3 ==
  Demux : Demux  Tag=STV Demux  Outputs=1
  FromWs : FromWorkspace  Tag=STV FromWs  VariableName=tuvar  SampleTime=0
      SigBuilderData=|
      | common.afterFinalStr = 'Extrapolate'
      | common.sampleTime = 0
      | dataSet(1).timeRange = [0 400]
      | dataSet(1).name = 'Group 1'
      | dataSet(2).timeRange = [0 400]
      | dataSet(2).name = 'Group 2'
      | sbobj.Groups(1).Name = 'Group 1'
      | sbobj.Groups(1).Signals.Name = 'PDR_ref'
      | sbobj.Groups(1).Signals.XData = [0 100 100 150 150 200 200 250 250 299 299 349.5 400]
      | sbobj.Groups(1).Signals.YData = [1.7 1.7 2.3 2.3 1.5 1.5 2 2 2.5 2.5 1.4 1.4 1.4]
      | sbobj.Groups(1).TimeRange = [0 400]
      | sbobj.Groups(2).Name = 'Group 2'
      | sbobj.Groups(2).Signals.Name = 'PDR_ref'
      | sbobj.Groups(2).Signals.XData = [0 400]
      | sbobj.Groups(2).Signals.YData = [0 0]
      | sbobj.Groups(2).TimeRange = [0 400]
  PDR_ref : Outport  Tag=STV Outport
  wires:
  FromWs/1 -> Demux/1
  Demux/1 -> PDR_ref/1

== system PECT08/Subsystem/Underflow valve step ==
  Demux : Demux  Tag=STV Demux  Outputs=1
  FromWs : FromWorkspace  Tag=STV FromWs  VariableName=tuvar  SampleTime=0
      SigBuilderData=|
      | common.afterFinalStr = 'Extrapolate'
      | common.sampleTime = 0
      | dataSet.timeRange = [0 1000]
      | dataSet.name = 'Group 1'
      | sbobj.Groups.Name = 'Group 1'
      | sbobj.Groups.Signals.Name = 'Signal 1'
      | sbobj.Groups.Signals.XData = [0 100 100 150 150 200 200 250 250 1000]
      | sbobj.Groups.Signals.YData = [0.7 0.7 0.45 0.45 0.6 0.6 0.4 0.4 0.5 0.5]
      | sbobj.Groups.TimeRange = [0 1000]
  Signal 1 : Outport  Tag=STV Outport
  wires:
  Demux/1 -> Signal 1/1
  FromWs/1 -> Demux/1

== system PECT08/Subsystem/Vu ==
  Demux : Demux  Tag=STV Demux  Outputs=1
  FromWs : FromWorkspace  Tag=STV FromWs  VariableName=tuvar  SampleTime=0
      SigBuilderData=|
      | common.afterFinalStr = 'Extrapolate'
      | common.sampleTime = 0
      | dataSet.timeRange = [0 1000]
      | dataSet.name = 'Group 1'
      | sbobj.Groups.Name = 'Group 1'
      | sbobj.Groups.Signals.Name = 'Signal 1'
      | sbobj.Groups.Signals.XData = [0 100 100 150 150 200 200 250 250 300 300 350 350 400 400 450 450 550 550 1000]
      | sbobj.Groups.Signals.YData = [0.37 0.37 0.45 0.45 0.7 0.7 0.4 0.4 1 1 0.6 0.6 0.37 0.37 0.8 0.8 0.6 0.6 0.4 0.4]
      | sbobj.Groups.TimeRange = [0 1000]
  Signal 1 : Outport  Tag=STV Outport
  wires:
  Demux/1 -> Signal 1/1
  FromWs/1 -> Demux/1

== system PECT08/Subsystem/underflow_valve_oscilation1 ==
  Demux : Demux  Tag=STV Demux  Outputs=3
  FromWs : FromWorkspace  Tag=STV FromWs  VariableName=tuvar  SampleTime=0
      SigBuilderData=|
      | common.afterFinalStr = 'Extrapolate'
      | common.sampleTime = 0
      | dataSet.timeRange = [0 1000]
      | dataSet.name = 'Group 1'
      | sbobj.Groups.Name = 'Group 1'
      | sbobj.Groups.Signals(1).Name = 'Signal 1'
      | sbobj.Groups.Signals(1).XData = [0 2.5 5 7.5 10 12.5 15 17.5 20 22.5 25 27.5 30 32.5 35 37.5 40 42.5 45 47.5 50 52.5 55 57.5 60 62.5 65 67.5 70 72.5 75 77.5 80 82.5 85 87.5 90 92.5 95 97.5 100 102.5 105 107.5 110 112.5 115 117.5 120 122.5 125 127.5 130 132.5 135 137.5 140 142.5 145 147.5 150 152.5 155 157.5 160 162.5 165 167.5 170 172.5 175 177.5 180 182.5 185 187.5 190 192.5 195 197.5 200 202.5 205 207.5 210 212.5 215 217.5 220 222.5 225 227.5 230 232.5 235 237.5 240 242.5 245 247.5 250 252.5 255 257.5 260 262.5 265 267.5 270 272.5 275 277.5 280 282.5 285 287.5 290 292.5 295 297.5 300 302.5 305 307.5 310 312.5 315 317.5 320 322.5 325 327.5 330 332.5 335 337.5 340 342.5 345 347.5 350 352.5 355 357.5 360 362.5 365 367.5 370 372.5 375 377.5 380 382.5 385 387.5 390 392.5 395 397.5 400 402.5 405 407.5 410 412.5 415 417.5 420 422.5 425 427.5 430 432.5 435 437.5 440 442.5 445 447.5 450 452.5 455 457.5 460 462.5 465 467.5 470 472.5 475 477.5 480 482.5 485 487.5 490 492.5 495 497.5 500 502.5 505 507.5 510 512.5 515 517.5 520 522.5 525 527.5 530 532.5 535 537.5 540 542.5 545 547.5 550 552.5 555 557.5 560 562.5 565 567.5 570 572.5 575 577.5 580 582.5 585 587.5 590 592.5 595 597.5 600 602.5 605 607.5 610 612.5 615 617.5 620 622.5 625 627.5 630 632.5 635 637.5 640 642.5 645 647.5 650 652.5 655 657.5 660 662.5 665 667.5 670 672.5 675 677.5 680 682.5 685 687.5 690 692.5 695 697.5 700 702.5 705 707.5 710 712.5 715 717.5 720 722.5 725 727.5 730 732.5 735 737.5 740 742.5 745 747.5 750 752.5 755 757.5 760 762.5 765 767.5 770 772.5 775 777.5 780 782.5 785 787.5 790 792.5 795 797.5 800 802.5 805 807.5 810 812.5 815 817.5 820 822.5 825 827.5 830 832.5 835 837.5 840 842.5 845 847.5 850 852.5 855 857.5 860 862.5 865 867.5 870 872.5 875 877.5 880 882.5 885 887.5 890 892.5 895 897.5 900 902.5 905 907.5 910 912.5 915 917.5 920 922.5 925 927.5 930 932.5 935 937.5 940 942.5 945 947.5 950 952.5 955 957.5 960 962.5 965 967.5 970 972.5 975 977.5 980 982.5 985 987.5 990 992.5 995 997.5 1000]
      | sbobj.Groups.Signals(1).YData = [0.42 0.441213203436 0.45 0.441213203436 0.42 0.398786796564 0.39 0.398786796564 0.42 0.441213203436 0.45 0.441213203436 ... (401 elements, 1x401)]
      | sbobj.Groups.Signals(2).Name = 'Signal 2'
      | sbobj.Groups.Signals(2).XData = [0 1.5873015873 3.1746031746 4.7619047619 6.34920634921 7.93650793651 9.52380952381 11.1111111111 12.6984126984 14.2857142857 15.873015873 17.4603174603 ... (632 elements, 1x632)]
      | sbobj.Groups.Signals(2).YData = [0.45 0.482139380484 0.499240387651 0.493301270189 0.467101007166 0.432898992834 0.406698729811 0.400759612349 0.417860619516 0.45 0.482139380484 0.499240387651 ... (632 elements, 1x632)]
      | sbobj.Groups.Signals(3).Name = 'Signal 3'
      | sbobj.Groups.Signals(3).XData = [0 3.7037037037 7.40740740741 11.1111111111 14.8148148148 18.5185185185 22.2222222222 25.9259259259 29.6296296296 33.3333333333 37.037037037 40.7407407407 ... (271 elements, 1x271)]
      | sbobj.Groups.Signals(3).YData = [0.45 0.482139380484 0.499240387651 0.493301270189 0.467101007166 0.432898992834 0.406698729811 0.400759612349 0.417860619516 0.45 0.482139380484 0.499240387651 ... (271 elements, 1x271)]
      | sbobj.Groups.TimeRange = [0 1000]
  Signal 1 : Outport  Tag=STV Outport
  Signal 2 : Outport  Tag=STV Outport  Port=2
  Signal 3 : Outport  Tag=STV Outport  Port=3
  wires:
  Demux/1 -> Signal 1/1
  FromWs/1 -> Demux/1
  Demux/2 -> Signal 2/1
  Demux/3 -> Signal 3/1

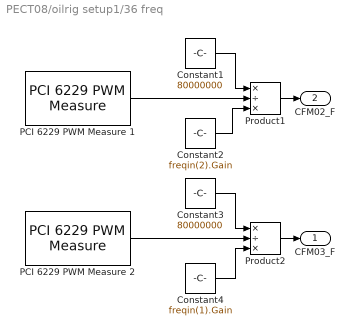
== system PECT08/oilrig setup1/36 freq ==
  Constant1 : Constant  Value=80000000
  Constant2 : Constant  Value=freqin(2).Gain
  Constant3 : Constant  Value=80000000
  Constant4 : Constant  Value=freqin(1).Gain
  PCI 6229 PWM Measure 1 : xpcnilib/Counter/M Series/PCI 6229 PWM Measure   channel=0  trigmd=Between Rising Edges  filter=None  tsamp=0.01  slot=[3,6]
  PCI 6229 PWM Measure 2 : xpcnilib/Counter/M Series/PCI 6229 PWM Measure   channel=1  trigmd=Between Rising Edges  filter=None  tsamp=0.01  slot=[3,6]
  Product1 : Product  Inputs=*/*
  Product2 : Product  Inputs=*/*
  CFM03_F : Outport
  CFM02_F : Outport  Port=2
  wires:
  PCI 6229 PWM Measure 1/1 -> Product1/2
  Constant1/1 -> Product1/1
  Product1/1 -> CFM02_F/1
  PCI 6229 PWM Measure 2/1 -> Product2/2
  Constant3/1 -> Product2/1
  Product2/1 -> CFM03_F/1
  Constant2/1 -> Product1/3
  Constant4/1 -> Product2/3

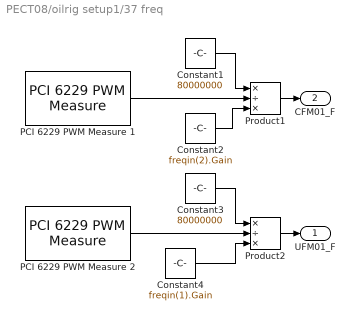
== system PECT08/oilrig setup1/37 freq ==
  Constant1 : Constant  Value=80000000
  Constant2 : Constant  Value=freqin(2).Gain
  Constant3 : Constant  Value=80000000
  Constant4 : Constant  Value=freqin(1).Gain
  PCI 6229 PWM Measure 1 : xpcnilib/Counter/M Series/PCI 6229 PWM Measure   channel=0  trigmd=Between Rising Edges  filter=None  tsamp=0.01  slot=[3,7]
  PCI 6229 PWM Measure 2 : xpcnilib/Counter/M Series/PCI 6229 PWM Measure   channel=1  trigmd=Between Rising Edges  filter=None  tsamp=0.01  slot=[3,7]
  Product1 : Product  Inputs=*/*
  Product2 : Product  Inputs=*/*
  UFM01_F : Outport
  CFM01_F : Outport  Port=2
  wires:
  PCI 6229 PWM Measure 1/1 -> Product1/2
  Constant1/1 -> Product1/1
  Product1/1 -> CFM01_F/1
  PCI 6229 PWM Measure 2/1 -> Product2/2
  Constant3/1 -> Product2/1
  Product2/1 -> UFM01_F/1
  Constant4/1 -> Product2/3
  Constant2/1 -> Product1/3

== system PECT08/oilrig setup1/PCI_6229_out1 ==
  ctrl : Inport
  DA_sink : xpcnilib/D//A/M Series/PCI-6229 DA  channel=[3 4]  reset=[1]  initValue=[0]  sampletime=0.01  slot=[3,5]
  gain : Constant  Value=gain
  offset : Constant  Value=offset
  transform : MATLAB Function  TreatAsAtomicUnit=on
  wires:
  transform/1(WP03) -> DA_sink/1
  transform/2(CV07) -> DA_sink/2
  ctrl/1 -> transform/1(u)
  gain/1 -> transform/2(gain)
  offset/1 -> transform/3(offset)

== system PECT08/oilrig setup1/PCI_6704_out ==
  ctrl : Inport
  DA_sink : xpcnilib/D//A/PCI-6704 DA  channel=[18 19 20 5 16 17 2 3 4 6 8 9 10 12 14 15]  sampletime=0.01  pcislot=[3,4]
  gain : Constant  Value=gain
  offset : Constant  Value=offset
  transform : MATLAB Function  TreatAsAtomicUnit=on
  wires:
  transform/1(OP01) -> DA_sink/1
  transform/2(OP02) -> DA_sink/2
  transform/3(OP03) -> DA_sink/3
  transform/4(WP01) -> DA_sink/4
  transform/5(WP02) -> DA_sink/5
  transform/6(OP04) -> DA_sink/6
  transform/7(AFM01) -> DA_sink/7
  transform/8(AFM02) -> DA_sink/8
  transform/9(AFM03) -> DA_sink/9
  transform/10(CV03) -> DA_sink/10
  transform/11(CV04) -> DA_sink/11
  transform/12(CV09) -> DA_sink/12
  transform/13(CV05) -> DA_sink/13
  transform/14(CV12) -> DA_sink/14
  transform/15(CV22) -> DA_sink/15
  transform/16(CV15) -> DA_sink/16
  ctrl/1 -> transform/1(u)
  gain/1 -> transform/2(gain)
  offset/1 -> transform/3(offset)

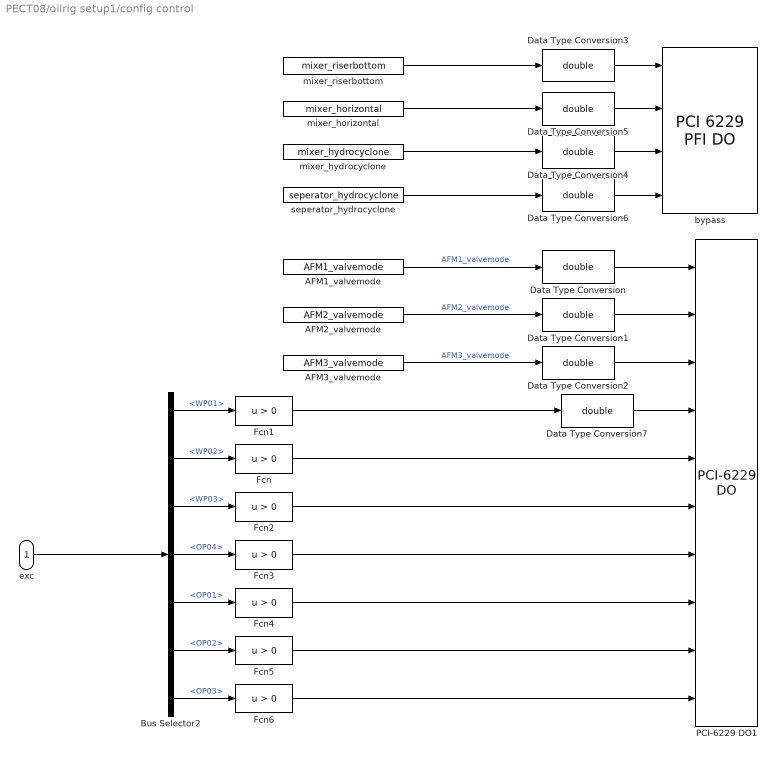
== system PECT08/oilrig setup1/config control ==
  exc : Inport
  AFM1_valvemode : Constant  Value=AFM1_valvemode
  AFM2_valvemode : Constant  Value=AFM2_valvemode
  AFM3_valvemode : Constant  Value=AFM3_valvemode
  Bus Selector2 : BusSelector  OutputSignals=WP01,WP02,WP03,OP04,OP01,OP02,OP03
  Data Type Conversion{,1..7} (8 alike) : DataTypeConversion  OutDataTypeStr=double
  Fcn{,1..6} (7 alike) : Fcn  Expr=u > 0
  PCI-6229 DO1 : xpcnilib/Digital Output/M Series/PCI-6229 DO  channel=[13 14 15 9 10 11 12 16 17 18]  reset=[1]  initValue=[1 1 1 0 0 0 0 0 0 0]  sampletime=0.01  slot=[3,5]
  bypass : xpcnilib/Digital Output/M Series/PCI 6229 PFI DO   channel=[0 1 2 3]  reset=0  initial=0  sampleTime=0.01  slot=[3,5]
  mixer_horizontal : Constant  Value=mixer_horizontal
  mixer_hydrocyclone : Constant  Value=mixer_hydrocyclone
  mixer_riserbottom : Constant  Value=mixer_riserbottom
  seperator_hydrocyclone : Constant  Value=seperator_hydrocyclone
  wires:
  Bus Selector2/2 -> Fcn/1  "<WP02>"
  exc/1 -> Bus Selector2/1
  Bus Selector2/1 -> Fcn1/1  "<WP01>"
  Bus Selector2/3 -> Fcn2/1  "<WP03>"
  Bus Selector2/4 -> Fcn3/1  "<OP04>"
  Fcn/1 -> PCI-6229 DO1/5
  Fcn2/1 -> PCI-6229 DO1/6
  Fcn3/1 -> PCI-6229 DO1/7
  Bus Selector2/5 -> Fcn4/1  "<OP01>"
  Bus Selector2/6 -> Fcn5/1  "<OP02>"
  Bus Selector2/7 -> Fcn6/1  "<OP03>"
  Fcn4/1 -> PCI-6229 DO1/8
  Fcn5/1 -> PCI-6229 DO1/9
  Fcn6/1 -> PCI-6229 DO1/10
  Data Type Conversion/1 -> PCI-6229 DO1/1
  Data Type Conversion2/1 -> PCI-6229 DO1/3
  Data Type Conversion1/1 -> PCI-6229 DO1/2
  Data Type Conversion3/1 -> bypass/1
  Data Type Conversion6/1 -> bypass/4
  Data Type Conversion5/1 -> bypass/2
  Data Type Conversion4/1 -> bypass/3
  Data Type Conversion7/1 -> PCI-6229 DO1/4
  Fcn1/1 -> Data Type Conversion7/1
  AFM1_valvemode/1 -> Data Type Conversion/1  "AFM1_valvemode"
  AFM2_valvemode/1 -> Data Type Conversion1/1  "AFM2_valvemode"
  AFM3_valvemode/1 -> Data Type Conversion2/1  "AFM3_valvemode"
  mixer_riserbottom/1 -> Data Type Conversion3/1
  mixer_horizontal/1 -> Data Type Conversion5/1
  mixer_hydrocyclone/1 -> Data Type Conversion4/1
  seperator_hydrocyclone/1 -> Data Type Conversion6/1

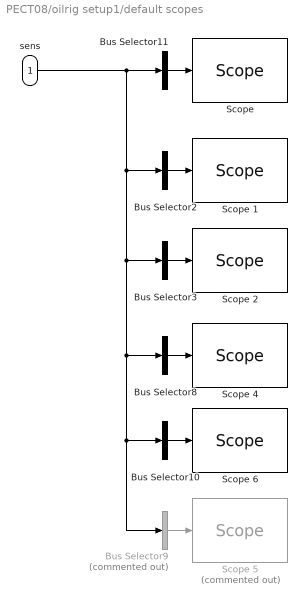
== system PECT08/oilrig setup1/default scopes ==
  sens : Inport
  Bus Selector10 : BusSelector  OutputSignals=PCI1.CV04,PCI1.CV09,signal2.PT02,signal2.PT03,signal3.PCI3.PT01,signal2.OIW01,signal2.OIW02,signal3.PCI3.MLT01_A,signal3.PCI3.LT02  OutputAsBus=on
  Bus Selector11 : BusSelector  OutputSignals=signal2.CFM03_F,signal2.CFM03_D,PCI1.CV03,signal2.PT14,signal2.MLT02_A,signal2.MLT02_B,signal2.DPT03,signal2.DPT04  OutputAsBus=on
  Bus Selector2 : BusSelector  OutputSignals=PCI1.CV15,signal3.PCI3.DPT02,signal3.PCI3.MFM04,PCI1.CV05,signal3.PCI3.PT11,signal3.PCI3.UFM01_D,signal3.PCI3.PT13,signal2.PT15,signal2.PT12  OutputAsBus=on
  Bus Selector3 : BusSelector  OutputSignals=signal3.PCI3.MFM02,signal2.MFM01,signal3.PCI3.MFM04,signal3.CFM02_F  OutputAsBus=on
  Bus Selector8 : BusSelector  OutputSignals=signal2.CFM03_F,signal3.CFM02_F,signal3.UFM01_F,signal3.CFM01_F  OutputAsBus=on
  Bus Selector9 : BusSelector  Commented=on  OutputSignals=signal2.PT05,signal2.TT06  OutputAsBus=on
  "Scope " : slrtlib/Displays and Logging/Scope   scopeno=10  scopetype=Target  autostart=on  viewmode=Numerical  formatstr='%15.6f'  grid=on  ylimits=[-1,1]  nosamples=25  noprepostsamples=0  interleave=1  triggermode=FreeRun  triggersignal=1  trigsignalfromport=off  triggerlevel=0.0  triggerslope=Either  triggerscope=1  triggersample=0  filename=data.dat  mode=Lazy  writesize=512  autorestart=off  dynamicfilemode=off  maxwritefilesize=512*1024^2
  Scope 1 : slrtlib/Displays and Logging/Scope   scopeno=11  scopetype=Target  autostart=on  viewmode=Numerical  formatstr='%15.6f'  grid=on  ylimits=[0,6]  nosamples=100  noprepostsamples=0  interleave=1  triggermode=FreeRun  triggersignal=1  trigsignalfromport=off  triggerlevel=0.0  triggerslope=Either  triggerscope=1  triggersample=0  filename=data.dat  mode=Lazy  writesize=512  autorestart=off  dynamicfilemode=off  maxwritefilesize=512*1024^2
  Scope 2 : slrtlib/Displays and Logging/Scope   scopeno=12  scopetype=Target  autostart=on  viewmode=Numerical  formatstr='%15.6f'  grid=on  ylimits=[0,6]  nosamples=25  noprepostsamples=0  interleave=1  triggermode=FreeRun  triggersignal=1  trigsignalfromport=off  triggerlevel=0.0  triggerslope=Either  triggerscope=1  triggersample=0  filename=data.dat  mode=Lazy  writesize=512  autorestart=off  dynamicfilemode=off  maxwritefilesize=512*1024^2
  Scope 4 : slrtlib/Displays and Logging/Scope   scopeno=13  scopetype=Target  autostart=on  viewmode=Numerical  formatstr='%15.6f L/s'  grid=on  ylimits=[0,2]  nosamples=25  noprepostsamples=0  interleave=1  triggermode=FreeRun  triggersignal=1  trigsignalfromport=off  triggerlevel=0.0  triggerslope=Either  triggerscope=1  triggersample=0  filename=data.dat  mode=Lazy  writesize=512  autorestart=off  dynamicfilemode=off  maxwritefilesize=512*1024^2
  Scope 5 : slrtlib/Displays and Logging/Scope   Commented=on  scopeno=6  scopetype=Target  autostart=on  viewmode=Numerical  formatstr='%15.6f'  grid=on  ylimits=[0,2]  nosamples=100  noprepostsamples=0  interleave=1  triggermode=FreeRun  triggersignal=1  trigsignalfromport=off  triggerlevel=0.0  triggerslope=Either  triggerscope=1  triggersample=0  filename=data.dat  mode=Lazy  writesize=512  autorestart=off  dynamicfilemode=off  maxwritefilesize=512*1024^2
  Scope 6 : slrtlib/Displays and Logging/Scope   scopeno=14  scopetype=Target  autostart=on  viewmode=Numerical  formatstr='%15.6f'  grid=on  ylimits=[0,2]  nosamples=100  noprepostsamples=0  interleave=1  triggermode=FreeRun  triggersignal=1  trigsignalfromport=off  triggerlevel=0.0  triggerslope=Either  triggerscope=1  triggersample=0  filename=data.dat  mode=Lazy  writesize=512  autorestart=off  dynamicfilemode=off  maxwritefilesize=512*1024^2
  wires:
  Bus Selector3/1 -> Scope 2/1
  Bus Selector2/1 -> Scope 1/1
  Bus Selector8/1 -> Scope 4/1
  Bus Selector9/1 -> Scope 5/1
  Bus Selector10/1 -> Scope 6/1
  sens/1 -> Bus Selector8/1, Bus Selector9/1, Bus Selector10/1, Bus Selector3/1, Bus Selector2/1, Bus Selector11/1
  Bus Selector11/1 -> "Scope "/1

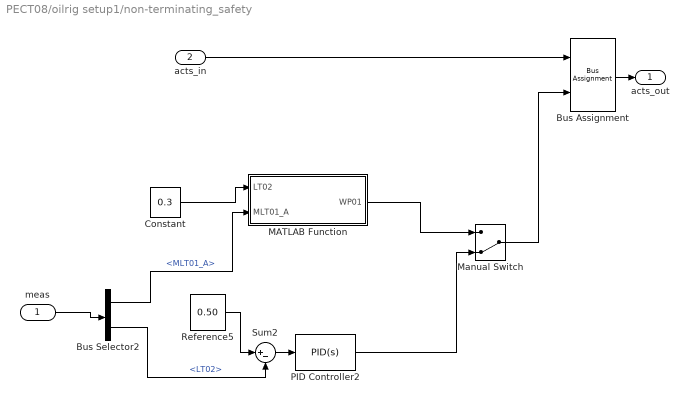
== system PECT08/oilrig setup1/non-terminating_safety ==
  meas : Inport
  acts_in : Inport  Port=2
  Bus Assignment : BusAssignment  AssignedSignals=WP01
  Bus Selector2 : BusSelector  OutputSignals=signal3.PCI3.MLT01_A,signal3.PCI3.LT02
  Constant : Constant  Value=0.3
  MATLAB Function : MATLAB Function  TreatAsAtomicUnit=on
  Manual Switch : ManualSwitch  CurrentSetting=0
  PID Controller2 : simulink/Continuous/PID Controller  Controller=PID  TimeDomain=Continuous-time  SampleTime=-1  IntegratorMethod=Forward Euler  FilterMethod=Forward Euler  Form=Parallel  UseFilter=on  ControllerParametersSource=internal  P=7.5  I=0  D=0  N=100  InitialConditionSource=internal  InitialConditionForIntegrator=0  InitialConditionForFilter=0  ExternalReset=none  LimitOutput=on  UpperSaturationLimit=1  LowerSaturationLimit=0  LinearizeAsGain=on  AntiWindupMode=clamping  Kb=1  TrackingMode=off  Kt=1  PParamMin=[]  PParamMax=[]  IParamMin=[]  IParamMax=[]  DParamMin=[]  DParamMax=[]  NParamMin=[]  NParamMax=[]  KbParamMin=[]  KbParamMax=[]  KtParamMin=[]  KtParamMax=[]  POutMin=[]  POutMax=[]  IOutMin=[]  IOutMax=[]  DOutMin=[]  DOutMax=[]  NOutMin=[]  NOutMax=[]  KbOutMin=[]  KbOutMax=[]  KtOutMin=[]  KtOutMax=[]  IntegratorOutMin=[]  IntegratorOutMax=[]  FilterOutMin=[]  FilterOutMax=[]  SumOutMin=[]  SumOutMax=[]  SumI1OutMin=[]  SumI1OutMax=[]  SumI2OutMin=[]  SumI2OutMax=[]  SumI3OutMin=[]  SumI3OutMax=[]  SumDOutMin=[]  SumDOutMax=[]  SaturationOutMin=[]  SaturationOutMax=[]  IntegratorContinuousStateAttributes=''  IntegratorStateMustResolveToSignalObject=off  IntegratorRTWStateStorageClass=Auto  FilterContinuousStateAttributes=''  FilterStateMustResolveToSignalObject=off  FilterRTWStateStorageClass=Auto  DifferentiatorICPrevScaledInput=0  DifferentiatorOutMin=[]  DifferentiatorOutMax=[]
  Reference5 : Constant  Value=0.50
  Sum2 : Sum  Inputs=|+-
  acts_out : Outport
  wires:
  Bus Assignment/1 -> acts_out/1
  meas/1 -> Bus Selector2/1
  Constant/1 -> MATLAB Function/1(LT02)
  Bus Selector2/1 -> MATLAB Function/2(MLT01_A)  "<MLT01_A>"
  acts_in/1 -> Bus Assignment/1
  Reference5/1 -> Sum2/1
  Sum2/1 -> PID Controller2/1
  PID Controller2/1 -> Manual Switch/2
  MATLAB Function/1(WP01) -> Manual Switch/1
  Manual Switch/1 -> Bus Assignment/2
  Bus Selector2/2 -> Sum2/2  "<LT02>"

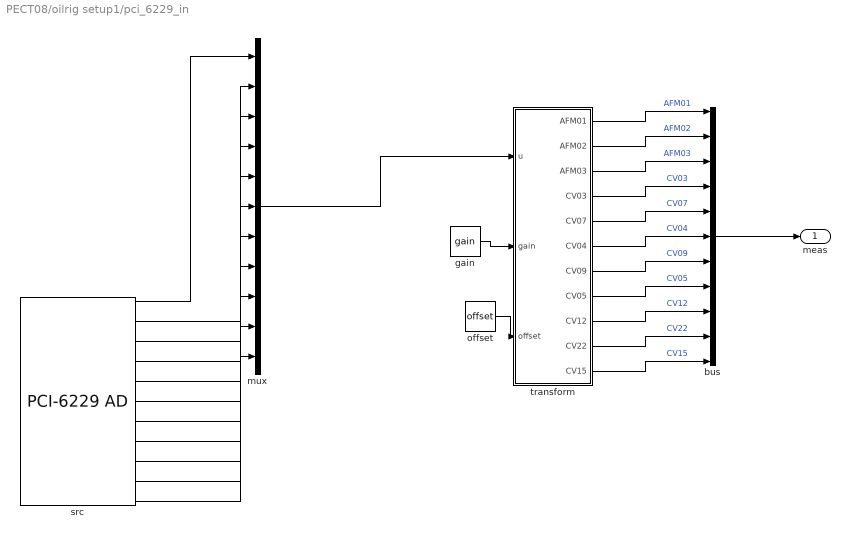
== system PECT08/oilrig setup1/pci_6229_in ==
  bus : BusCreator  Inputs=11
  gain : Constant  Value=gain
  mux : Mux  Inputs=11
  offset : Constant  Value=offset
  src : xpcnilib/A//D/M Series/PCI-6229 AD  channel=[9 2 10 11 4 12 5 13 14 15 8]  range=[10]  coupling=[0]  scantime=5e-6  sampletime=0.01  slot=[3,5]
  transform : MATLAB Function  TreatAsAtomicUnit=on
  meas : Outport
  wires:
  src/1 -> mux/1
  transform/1(AFM01) -> bus/1  "AFM01"
  src/2 -> mux/2
  transform/2(AFM02) -> bus/2  "AFM02"
  src/3 -> mux/3
  transform/3(AFM03) -> bus/3  "AFM03"
  src/4 -> mux/4
  transform/4(CV03) -> bus/4  "CV03"
  src/5 -> mux/5
  transform/5(CV07) -> bus/5  "CV07"
  src/6 -> mux/6
  transform/6(CV04) -> bus/6  "CV04"
  src/7 -> mux/7
  transform/7(CV09) -> bus/7  "CV09"
  src/8 -> mux/8
  transform/8(CV05) -> bus/8  "CV05"
  src/9 -> mux/9
  transform/9(CV12) -> bus/9  "CV12"
  src/10 -> mux/10
  transform/10(CV22) -> bus/10  "CV22"
  src/11 -> mux/11
  transform/11(CV15) -> bus/11  "CV15"
  mux/1 -> transform/1(u)
  gain/1 -> transform/2(gain)
  offset/1 -> transform/3(offset)
  bus/1 -> meas/1

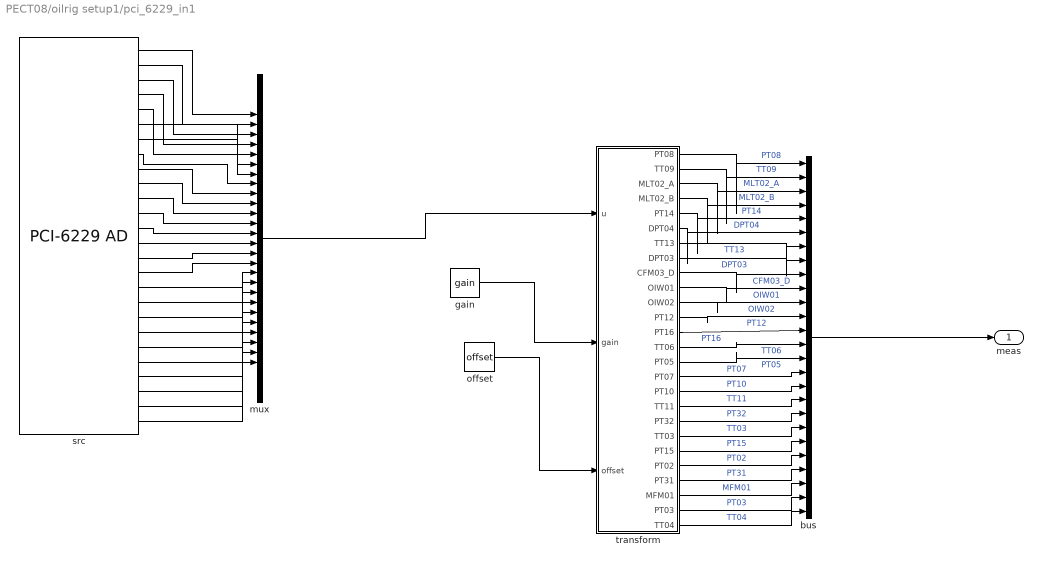
== system PECT08/oilrig setup1/pci_6229_in1 ==
  bus : BusCreator  Inputs=26
  gain : Constant  Value=gain
  mux : Mux  Inputs=26
  offset : Constant  Value=offset
  src : xpcnilib/A//D/M Series/PCI-6229 AD  channel=[24 31 23 30 22 29 21 28 20 27 19 8 15 7 14 6 13 5 12 4 11 3 10 2 9 1]  range=[10]  coupling=[0]  scantime=5e-6  sampletime=0.01  slot=[3,6]
  transform : MATLAB Function  TreatAsAtomicUnit=on
  meas : Outport
  wires:
  src/1 -> mux/1
  transform/1(PT08) -> bus/1  "PT08"
  src/2 -> mux/2
  transform/2(TT09) -> bus/2  "TT09"
  src/3 -> mux/3
  transform/3(MLT02_A) -> bus/3  "MLT02_A"
  src/4 -> mux/4
  transform/4(MLT02_B) -> bus/4  "MLT02_B"
  src/5 -> mux/5
  transform/5(PT14) -> bus/5  "PT14"
  src/6 -> mux/6
  transform/6(DPT04) -> bus/6  "DPT04"
  src/7 -> mux/7
  transform/7(TT13) -> bus/7  "TT13"
  src/8 -> mux/8
  transform/8(DPT03) -> bus/8  "DPT03"
  src/9 -> mux/9
  transform/9(CFM03_D) -> bus/9  "CFM03_D"
  src/10 -> mux/10
  transform/10(OIW01) -> bus/10  "OIW01"
  src/11 -> mux/11
  transform/11(OIW02) -> bus/11  "OIW02"
  src/12 -> mux/12
  transform/12(PT12) -> bus/12  "PT12"
  src/13 -> mux/13
  transform/13(PT16) -> bus/13  "PT16"
  src/14 -> mux/14
  transform/14(TT06) -> bus/14  "TT06"
  src/15 -> mux/15
  transform/15(PT05) -> bus/15  "PT05"
  src/16 -> mux/16
  transform/16(PT07) -> bus/16  "PT07"
  src/17 -> mux/17
  transform/17(PT10) -> bus/17  "PT10"
  src/18 -> mux/18
  transform/18(TT11) -> bus/18  "TT11"
  src/19 -> mux/19
  transform/19(PT32) -> bus/19  "PT32"
  src/20 -> mux/20
  transform/20(TT03) -> bus/20  "TT03"
  src/21 -> mux/21
  transform/21(PT15) -> bus/21  "PT15"
  src/22 -> mux/22
  transform/22(PT02) -> bus/22  "PT02"
  src/23 -> mux/23
  transform/23(PT31) -> bus/23  "PT31"
  src/24 -> mux/24
  transform/24(MFM01) -> bus/24  "MFM01"
  src/25 -> mux/25
  transform/25(PT03) -> bus/25  "PT03"
  src/26 -> mux/26
  transform/26(TT04) -> bus/26  "TT04"
  mux/1 -> transform/1(u)
  gain/1 -> transform/2(gain)
  offset/1 -> transform/3(offset)
  bus/1 -> meas/1

== system PECT08/oilrig setup1/pci_6229_in2 ==
  bus : BusCreator  Inputs=16
  gain : Constant  Value=gain
  mux : Mux  Inputs=16
  offset : Constant  Value=offset
  src : xpcnilib/A//D/M Series/PCI-6229 AD  channel=[24 31 23 30 22 29 21 28 20 27 19 26 18 17 8 15]  range=[10]  coupling=[0]  scantime=5e-6  sampletime=0.01  slot=[3,7]
  transform : MATLAB Function  TreatAsAtomicUnit=on
  meas : Outport
  wires:
  src/1 -> mux/1
  transform/1(MLT01_A) -> bus/1  "MLT01_A"
  src/2 -> mux/2
  transform/2(MLT01_B) -> bus/2  "MLT01_B"
  src/3 -> mux/3
  transform/3(LT02) -> bus/3  "LT02"
  src/4 -> mux/4
  transform/4(TT05) -> bus/4  "TT05"
  src/5 -> mux/5
  transform/5(LT01) -> bus/5  "LT01"
  src/6 -> mux/6
  transform/6(TT12) -> bus/6  "TT12"
  src/7 -> mux/7
  transform/7(PT13) -> bus/7  "PT13"
  src/8 -> mux/8
  transform/8(MFM02) -> bus/8  "MFM02"
  src/9 -> mux/9
  transform/9(PT11) -> bus/9  "PT11"
  src/10 -> mux/10
  transform/10(DPT02) -> bus/10  "DPT02"
  src/11 -> mux/11
  transform/11(PT01) -> bus/11  "PT01"
  src/12 -> mux/12
  transform/12(MFM04) -> bus/12  "MFM04"
  src/13 -> mux/13
  transform/13(TT01) -> bus/13  "TT01"
  src/14 -> mux/14
  transform/14(CFM02_D) -> bus/14  "CFM02_D"
  src/15 -> mux/15
  transform/15(UFM01_D) -> bus/15  "UFM01_D"
  src/16 -> mux/16
  transform/16(CFM01_D) -> bus/16  "CFM01_D"
  mux/1 -> transform/1(u)
  gain/1 -> transform/2(gain)
  offset/1 -> transform/3(offset)
  bus/1 -> meas/1

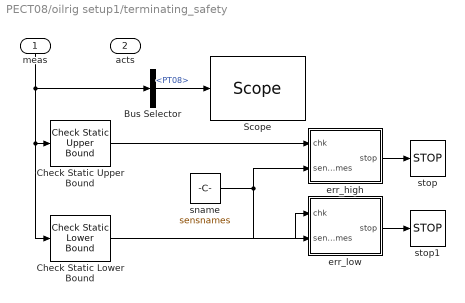
== system PECT08/oilrig setup1/terminating_safety ==
  meas : Inport
  acts : Inport  Port=2
  Bus Selector : BusSelector  OutputSignals=signal2.PT08
  Check Static Lower Bound : simulink/Model Verification/Check Static  Lower Bound  Description=[sensors.MinOp]-([sensors.MaxOp]-[sensors.MinOp])*0.05 <= u  min=[sensors.MinOp]-([sensors.MaxOp]-[sensors.MinOp])*0.05  min_included=on  enabled=on  stopWhenAssertionFail=off  export=on  icon=graphic
  Check Static Upper Bound : simulink/Model Verification/Check Static  Upper Bound  Description=u <= [sensors.MaxOp]+([sensors.MaxOp]-[sensors.MinOp])*0.05  max=[sensors.MaxOp]+([sensors.MaxOp]-[sensors.MinOp])*0.05  max_included=on  enabled=on  stopWhenAssertionFail=off  export=on  icon=graphic
  "Scope " : slrtlib/Displays and Logging/Scope   scopeno=15  scopetype=Target  autostart=on  viewmode=Graphical redraw  formatstr='%15.6f'  grid=on  ylimits=[0,0]  nosamples=250  noprepostsamples=0  interleave=1  triggermode=FreeRun  triggersignal=1  trigsignalfromport=off  triggerlevel=0.0  triggerslope=Either  triggerscope=1  triggersample=0  filename=data.dat  mode=Lazy  writesize=512  autorestart=off  dynamicfilemode=off  maxwritefilesize=512*1024^2
  err_high : MATLAB Function  TreatAsAtomicUnit=on
  err_low : MATLAB Function  TreatAsAtomicUnit=on
  sname : Constant  Value=sensnames
  stop : Stop
  stop1 : Stop
  wires:
  Check Static Upper Bound/1 -> err_high/1(chk)
  Check Static Lower Bound/1 -> err_low/1(chk)
  sname/1 -> err_high/2(sensnames), err_low/2(sensnames)
  err_high/1(stop) -> stop/1
  err_low/1(stop) -> stop1/1
  meas/1 -> Bus Selector/1, Check Static Lower Bound/1, Check Static Upper Bound/1
  Bus Selector/1 -> "Scope "/1  "<PT08>"

== system PECT08/oilrig setup1/to_logging_data ==
  meas : Inport
  "Scope " : slrtlib/Displays and Logging/Scope   scopeno=1  scopetype=Host  autostart=on  viewmode=Graphical redraw  formatstr='%15.6f'  grid=on  ylimits=[0,0]  nosamples=250  noprepostsamples=0  interleave=1  triggermode=FreeRun  triggersignal=1  trigsignalfromport=off  triggerlevel=0.0  triggerslope=Either  triggerscope=1  triggersample=0  filename=data.dat  mode=Lazy  writesize=512  autorestart=off  dynamicfilemode=off  maxwritefilesize=512*1024^2
  wires:
  meas/1 -> "Scope "/1

== system PECT08/oilrig setup1/to_logging_exc ==
  exc : Inport
  IC : InitialCondition  Value=zeros(numel(actuators),1)
  "Scope " : slrtlib/Displays and Logging/Scope   scopeno=2  scopetype=Host  autostart=on  viewmode=Graphical redraw  formatstr='%15.6f'  grid=on  ylimits=[0,0]  nosamples=250  noprepostsamples=0  interleave=1  triggermode=FreeRun  triggersignal=1  trigsignalfromport=off  triggerlevel=0.0  triggerslope=Either  triggerscope=1  triggersample=0  filename=data.dat  mode=Lazy  writesize=512  autorestart=off  dynamicfilemode=off  maxwritefilesize=512*1024^2
  wires:
  IC/1 -> "Scope "/1
  exc/1 -> IC/1

== matlab function PECT08/MATLAB Function1 ==
  data: Pi input; PDR output; Po input; Pu input
function PDR = fcn(Pi,Po,Pu)
%#codegen

PDR = (Pi-Po)/(Pi-Pu);

== matlab function PECT08/Subsystem/MATLAB Function ==
  data: Pi input; PDR output; Po input; Pu input
function PDR = fcn(Pi,Po,Pu)
%#codegen

PDR = (Pi-Po)/(Pi-Pu);

== matlab function PECT08/Subsystem/MATLAB Function1 ==
  data: u input; y output
function y = fcn(u)
%#codegen

y = 1-u;

== matlab function PECT08/MATLAB Function ==
  data: Pi input; PDR output; Po input; Pu input
function PDR = fcn(Pi,Po,Pu)
%#codegen

PDR = (Pi-Po)/(Pi-Pu);

== matlab function PECT08/oilrig setup1/PCI_6229_out1/transform ==
  data: WP03 output; u input; gain input; offset input; CV07 output
function [WP03,CV07]  = fcn(u,gain,offset)
   y = u.*gain-offset;
WP03 = y(1);
CV07 = y(2);

== matlab function PECT08/oilrig setup1/PCI_6704_out/transform ==
  data: OP01 output; OP02 output; u input; gain input; offset input; OP03 output; WP01 output; WP02 output; OP04 output; AFM01 output; AFM02 output; AFM03 output; CV03 output; CV04 output; CV09 output; CV05 output; CV12 output; CV22 output; CV15 output
function [OP01,OP02,OP03,WP01,WP02,OP04,AFM01,AFM02,AFM03,CV03,CV04,CV09,CV05,CV12,CV22,CV15]  = fcn(u,gain,offset)
   y = u.*gain-offset;
OP01 = y(1);
OP02 = y(2);
OP03 = y(3);
WP01 = y(4);
WP02 = y(5);
OP04 = y(6);
AFM01 = y(7);
AFM02 = y(8);
AFM03 = y(9);
CV03 = y(10);
CV04 = y(11);
CV09 = y(12);
CV05 = y(13);
CV12 = y(14);
CV22 = y(15);
CV15 = y(16);

== matlab function PECT08/oilrig setup1/non-terminating_safety/MATLAB Function ==
  data: LT02 input; WP01 output; MLT01_A input
function WP01 = fcn(LT02, MLT01_A)
%#codegen
persistent filling

if isempty(filling)
   filling = 0;
end

if (LT02 < 0.4) && (MLT01_A > 0.6)
   filling = 1;
end

if (LT02 > 0.6) || (MLT01_A < 0.5)
   filling = 0; 
end

WP01 = filling;

== matlab function PECT08/oilrig setup1/pci_6229_in/transform ==
  data: AFM01 output; AFM02 output; AFM03 output; CV03 output; CV07 output; CV04 output; CV09 output; CV05 output; u input; CV12 output; gain input; offset input; CV22 output; CV15 output
function [AFM01,AFM02,AFM03,CV03,CV07,CV04,CV09,CV05,CV12,CV22,CV15]  = fcn(u,gain,offset)
   y = u.*gain-offset;
AFM01 = y(1);
AFM02 = y(2);
AFM03 = y(3);
CV03 = y(4);
CV07 = y(5);
CV04 = y(6);
CV09 = y(7);
CV05 = y(8);
CV12 = y(9);
CV22 = y(10);
CV15 = y(11);

== matlab function PECT08/oilrig setup1/pci_6229_in1/transform ==
  data: PT08 output; TT09 output; u input; MLT02_A output; MLT02_B output; PT14 output; DPT04 output; TT13 output; DPT03 output; CFM03_D output; OIW01 output; OIW02 output; PT12 output; PT16 output; TT06 output; PT05 output; PT07 output; PT10 output; TT11 output; PT32 output; gain input; offset input; TT03 output; PT15 output; PT02 output; PT31 output; MFM01 output; PT03 output; TT04 output
function [PT08,TT09,MLT02_A,MLT02_B,PT14,DPT04,TT13,DPT03,CFM03_D,OIW01,OIW02,PT12,PT16,TT06,PT05,PT07,PT10,TT11,PT32,TT03,PT15,PT02,PT31,MFM01,PT03,TT04]  = fcn(u,gain,offset)
   y = u.*gain-offset;
PT08 = y(1);
TT09 = y(2);
MLT02_A = y(3);
MLT02_B = y(4);
PT14 = y(5);
DPT04 = y(6);
TT13 = y(7);
DPT03 = y(8);
CFM03_D = y(9);
OIW01 = y(10);
OIW02 = y(11);
PT12 = y(12);
PT16 = y(13);
TT06 = y(14);
PT05 = y(15);
PT07 = y(16);
PT10 = y(17);
TT11 = y(18);
PT32 = y(19);
TT03 = y(20);
PT15 = y(21);
PT02 = y(22);
PT31 = y(23);
MFM01 = y(24);
PT03 = y(25);
TT04 = y(26);

== matlab function PECT08/oilrig setup1/pci_6229_in2/transform ==
  data: MLT01_A output; MLT01_B output; LT02 output; u input; TT05 output; LT01 output; gain input; offset input; TT12 output; PT13 output; MFM02 output; PT11 output; DPT02 output; PT01 output; MFM04 output; TT01 output; CFM02_D output; UFM01_D output; CFM01_D output
function [MLT01_A,MLT01_B,LT02,TT05,LT01,TT12,PT13,MFM02,PT11,DPT02,PT01,MFM04,TT01,CFM02_D,UFM01_D,CFM01_D]  = fcn(u,gain,offset)
   y = u.*gain-offset;
MLT01_A = y(1);
MLT01_B = y(2);
LT02 = y(3);
TT05 = y(4);
LT01 = y(5);
TT12 = y(6);
PT13 = y(7);
MFM02 = y(8);
PT11 = y(9);
DPT02 = y(10);
PT01 = y(11);
MFM04 = y(12);
TT01 = y(13);
CFM02_D = y(14);
UFM01_D = y(15);
CFM01_D = y(16);

== matlab function PECT08/oilrig setup1/terminating_safety/err_high ==
  data: chk input; sensnames input uint8; stop output
function stop  = fcn(chk, sensnames)
%#codegen
%test = char(sensnames.');
test = sensnames.';
k = find(test == 47);
k = [0 k];
k = [k numel(test)];
stop = 0;
for i = 1:numel(chk)
    if chk(i) == 0
        str = char(test(k(i)+1:k(i+1)-1));
        Error = [str ': VALUE TOO HIGH ']
        coder.ceval('printf', ['%s' 10 0], Error);
        stop = stop+1;
    end
end
